simulink model "prMotor"  (R2021a)
settings: Solver=ode3  StartTime=0.0  StopTime=2  FixedStep=0.000125  RelTol=1e-3  EnableMultiTasking=on
values from neighbouring files (symbols this model uses):
  DELTA_EMF = 14    [prMotor_init.m]
  DELTA_THETA = 29    [prMotor_init.m]
  DT_GAIN = 102    [prMotor_init.m]
  DT_IREF_LIM = 205    [prMotor_init.m]
  DT_SET_H = 10    [prMotor_init.m]
  DT_SET_L = -10    [prMotor_init.m]
  DT_VALUE = 2    [prMotor_init.m]
  DUTY = 2048    [prMotor_init.m]
  DUTY_50 = 1024    [prMotor_init.m]
  EMF_GAIN = 759    [prMotor_init.m]
  ID_GAIN = 350    [prMotor_init.m]
  ID_LIM = 205    [prMotor_init.m]
  ID_RPM = 1800    [prMotor_init.m]
  IREF_FLT_A1 = -446    [prMotor_init.m]
  IREF_FLT_B0 = 289    [prMotor_init.m]
  IREF_FLT_B1 = 289    [prMotor_init.m]
  Ki = 0.048828125    [prMotor_init.m]
  mp_emf = [0	3	5	8	10	13	15	18	21	23	26	28	31	33	36	39	41	44	46	49	51	54	56	59	62	64	67	69	72	74	77	79	82	84	87	89	92	94	97	99	102	104	107	109	112	114	117	119	122	124	127	129	132	134	136	139	141	144	146	149	151	153	156	158	161	163	165	168	170	172	175	177	179	182	184	186	189	191	193	195	198	200	202	204	207	209	211	213	216	218	220	222	224	227	229	231	233	235	237	239	242	244	246	248	250	252	254	256	258	260	262 ...(+4035 chars)    [prMotor_init.m]
  mp_sin = [0	6	13	19	25	31	38	44	50	57	63	69	75	82	88	94	100	107	113	119	125	132	138	144	150	156	163	169	175	181	187	194	200	206	212	218	224	230	237	243	249	255	261	267	273	279	285	291	297	303	309	315	321	327	333	339	345	351	357	363	369	374	380	386	392	398	403	409	415	421	426	432	438	443	449	455	460	466	472	477	483	488	494	499	505	510	516	521	526	532	537	543	548	553	558	564	569	574	579	584	590	595	600	605	6 ...(+4281 chars)    [prMotor_init.m]
  mp_theta = [0	1	2	3	4	5	6	7	8	9	10	11	12	13	14	15	16	17	18	19	20	21	22	23	24	25	26	27	28	29	30	31	32	33	34	35	36	37	38	39	40	41	42	43	44	45	46	47	48	49	50	51	52	53	54	55	56	57	58	59	60	61	62	63	64	65	66	67	68	69	70	71	72	73	74	75	76	77	78	79	80	81	82	83	84	85	86	87	88	89	90	91	92	93	94	95	96	97	98	99	100	101	102	103	104	105	106	107	108	109	110	111	112	113	114	115	116	117	118	119	120	121	122	123	124	125	126	1 ...(+3610 chars)    [prMotor_init.m]
  PI_A1 = -1024    [prMotor_init.m]
  PI_B0 = 292    [prMotor_init.m]
  PI_B1 = -279    [prMotor_init.m]
  RPM_GAIN = 15000    [prMotor_init.m]
  RPM_LIM = 3000    [prMotor_init.m]
  RPM_LPF_A1 = -984    [prMotor_init.m]
  RPM_LPF_B0 = 20    [prMotor_init.m]
  RPM_LPF_B1 = 20    [prMotor_init.m]
  T_smp = 0.000125    [prMotor_init.m]
  THETA_ADV_LIM = 85    [prMotor_init.m]
libraries: simulink x1
(part 2 of 2)

== system prMotor/blm_curr_mdl_dec/FB_calc_dec/PI_calc_dec/PI_cont_b ==
  In : Inport
  Add : Sum
  PI_A1 : Gain  Gain=PI_A1
  PI_B0 : Gain  Gain=PI_B0
  PI_B1 : Gain  Gain=PI_B1
  Quantizer : Quantizer  QuantizationInterval=1
  Quantizer1 : Quantizer  QuantizationInterval=1
  Scale_2_10_a : Gain  Gain=2^-10
  Scale_2_10_b : Gain  Gain=2^-10
  Sub : Sum  Inputs=+-
  delay : Delay  DelayLength=1  InitialCondition=T_smp
  Out : Outport
  wires:
  Quantizer1/1 -> Sub/2
  Quantizer/1 -> Out/1
  Scale_2_10_a/1 -> Quantizer1/1
  Scale_2_10_b/1 -> Quantizer/1
  PI_A1/1 -> Scale_2_10_a/1
  PI_B1/1 -> Add/2
  PI_B0/1 -> Add/1
  Add/1 -> Scale_2_10_b/1
  Sub/1 -> PI_B0/1, delay/1
  In/1 -> Sub/1
  delay/1 -> PI_A1/1, PI_B1/1

== system prMotor/blm_curr_mdl_dec/FB_calc_dec/PI_calc_dec/PI_cont_c ==
  In : Inport
  Add : Sum
  PI_A1 : Gain  Gain=PI_A1
  PI_B0 : Gain  Gain=PI_B0
  PI_B1 : Gain  Gain=PI_B1
  Quantizer : Quantizer  QuantizationInterval=1
  Quantizer1 : Quantizer  QuantizationInterval=1
  Scale_2_10_a : Gain  Gain=2^-10
  Scale_2_10_b : Gain  Gain=2^-10
  Sub : Sum  Inputs=+-
  delay : Delay  DelayLength=1  InitialCondition=T_smp
  Out : Outport
  wires:
  Quantizer1/1 -> Sub/2
  Quantizer/1 -> Out/1
  Scale_2_10_a/1 -> Quantizer1/1
  Scale_2_10_b/1 -> Quantizer/1
  PI_A1/1 -> Scale_2_10_a/1
  PI_B1/1 -> Add/2
  PI_B0/1 -> Add/1
  Add/1 -> Scale_2_10_b/1
  Sub/1 -> PI_B0/1, delay/1
  In/1 -> Sub/1
  delay/1 -> PI_A1/1, PI_B1/1
